simulink model "Lights_harness"  (Simulink 7.7)
settings: Solver=FixedStepDiscrete  SolverMode=SingleTasking  StartTime=0.0  StopTime=100  FixedStep=.01  RelTol=1e-3
PostLoadFcn:
  | cd '..';
  | PostLoadFcn;
  | cd 'harness';
InitFcn:
  | if signalbuilder('Lights_harness/Signal Builder','activegroup') == 1
  |   CD_LIGHTS_FUNCTION.DataType = 'uint8';
  |   CD_LIGHTS_FUNCTION.Value = 255;
  |   CD_LIGHTS_FEEDBACK_FUNCTION.DataType = 'uint8';
  |   CD_LIGHTS_FEEDBACK_FUNCTION.Value = 255;
  | else
  |   CD_LIGHTS_FUNCTION.DataType = 'uint8';
  |   CD_LIGHTS_FUNCTION.Value = 0;
  |   CD_LIGHTS_FEEDBACK_FUNCTION.DataType = 'uint8';
  |   CD_LIGHTS_FEEDBACK_FUNCTION.Value = 0;
  | end
undefined symbols (not defined in the file): ACTIVE, INACTIVE, LIGHT_BUTTON_MASK, LIGHT_BUTTON_PRESS, LOW, NO_COMMUNICATION, NON_FUNCTIONAL, NORMAL, OORL, sigbuilder_block, srate100
libraries: simulink x2, MX_Library x1
settings Model: Creator=smindema  LastModifiedBy=aliebel  CovMetricSettings=dcmw  CovHTMLOptions=-aTS=1 -bRG=1 -bTC=1 -hTR=0 -nFC=0 -scm=1 -bcm=1 -xEv=0  covSaveCumulativeToWorkspaceVar=off  CovSaveSingleToWorkspaceVar=off
settings MATStruct: SampleTime=0.01  Offset=0  Priority=[1.0]
settings DataIOCC: LimitDataPoints=off  SaveOutput=off  SaveTime=off
settings OptimizationCC: BlockReduction=off  InlineParams=on  ExpressionFolding=off  StateBitsets=on  DataBitsets=on  UseTempVars=on  InitFltsAndDblsToZero=on  NoFixptDivByZeroProtection=on  EfficientFloat2IntCast=on  OptimizeModelRefInitCode=on
settings DebuggingCC: SaveWithParameterizedLinksMsg=none  MultiTaskDSMMsg=warning  MultiTaskCondExecSysMsg=none  IntegerOverflowMsg=none  ModelReferenceCSMismatchMessage=warning
settings HardwareCC: ProdBitPerInt=16  ProdBitPerPointer=16  ProdIntDivRoundTo=Floor  ProdEndianess=BigEndian  ProdWordSize=16  ProdHWDeviceType=Motorola HC12
settings ModelReferenceCC: ModelReferenceNumInstancesAllowed=Single
settings RTWCC: SystemTargetFile=ert.tlc  GenCodeOnly=on  TemplateMakefile=ert_default_tmf  Description=Real-Time Workshop Embedded Coder (no auto configuration)  GenerateReport=on  RetainRTWFile=on  ProcessScript=ert_make_rtw_hook  IncludeHyperlinkInReport=on  LaunchReport=on  IncludeERTFirstTime=on
settings RTWCC: CustomHeaderCode=|
  | #include "cpp_req_defines.h"
  | #include "hw_fin.h"
  | #include "cdata.h"
settings CodeAppCC: IgnoreCustomStorageClasses=off  DefineNamingRule=UpperCase
settings ERTTargetCC: TargetFcnLib=ansi_tfl_tmw.mat  FunctionExecutionProfile=off  MultiwordLength=2048  GenerateSampleERTMain=on  IncludeMdlTerminateFcn=off  SupportAbsoluteTime=off  SupportNonFinite=off  SupportComplex=off  PurelyIntegerCode=on  ERTCustomFileTemplate=gen_rtw_req_defines_h.tlc  GlobalDataDefinition=InSeparateSourceFile  GlobalDataReference=InSeparateHeaderFile  ConvertIfToSwitch=off

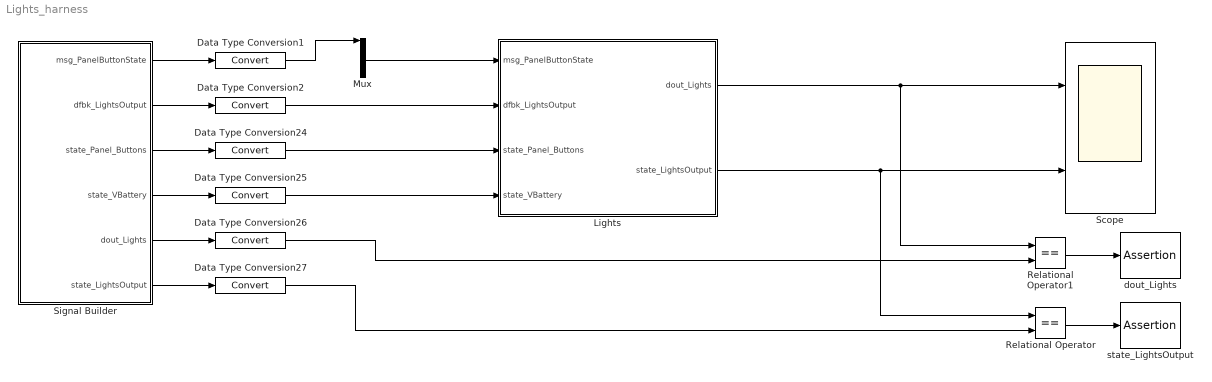
== system Lights_harness ==
  Data Type Conversion{1..2,24..27} (6 alike) : DataTypeConversion
  Lights : Subsystem  TreatAsAtomicUnit=on  SystemSampleTime=srate100  RTWFileName=mod_Outputs
      settings: RTWSystemCode=Function  RTWFileNameOpts=User specified
  Mux : Mux  Inputs=8
  Relational Operator : RelationalOperator  Operator===  OutDataTypeStr=boolean
  Relational Operator1 : RelationalOperator  Operator===  OutDataTypeStr=boolean
  Scope : Scope  NumInputPorts=2
      settings: TimeRange=100  YMin=0~0  YMax=6~10  DataFormat=Array
  Signal Builder : Subsystem  Tag=STV Subsys  LoadFcn=sigbuilder_block('load');  StartFcn=sigbuilder_block('start');  StopFcn=sigbuilder_block('stop');  ClipboardFcn=sigbuilder_block('clipboard');  mask(Sigbuilder block){}
      mask help: Create and generate interchangeable groups of signals whose waveforms are piecewise linear.
      mask init:
      | if ~strcmp(get_param(bdroot(gcbh),'SimulationStatus'),'stopped') tuvar = sigbuilder_block('maskInit'); end
      settings: CopyFcn=sigbuilder_block('copy');  DeleteFcn=sigbuilder_block('delete');  ModelCloseFcn=sigbuilder_block('modelClose');  PreSaveFcn=sigbuilder_block('preSave');  NameChangeFcn=sigbuilder_block('namechange');  OpenFcn=sigbuilder_block('open',[294.75 262.5 911.25 399.75 ]);  CloseFcn=sigbuilder_block('close');
      mask Display: plot(0, 0, 100, 100,[2, 2, 32, 32, 2], [68, 8, 8, 68, 68],[32, 2], [38, 38], [32, 19, 2],[53, 60, 44], [32, 17, 17, 2],[16, 16, 31, 31]);txt = getActiveGroup(gcbh);text(2, 100, txt,'verticalAlignment', 'top');
  dout_Lights : Assertion  Enabled=off
  state_LightsOutput : Assertion  Enabled=off
  wires:
  Relational Operator/1 -> state_LightsOutput/1
  Relational Operator1/1 -> dout_Lights/1
  Data Type Conversion26/1 -> Relational Operator1/2
  Data Type Conversion27/1 -> Relational Operator/2
  Lights/1(dout_Lights) -> Scope/1, Relational Operator1/1
  Lights/2(state_LightsOutput) -> Scope/2, Relational Operator/1
  Data Type Conversion2/1 -> Lights/2(dfbk_LightsOutput)
  Data Type Conversion24/1 -> Lights/3(state_Panel_Buttons)
  Data Type Conversion25/1 -> Lights/4(state_VBattery)
  Signal Builder/1(msg_PanelButtonState) -> Data Type Conversion1/1
  Signal Builder/2(dfbk_LightsOutput) -> Data Type Conversion2/1
  Signal Builder/3(state_Panel_Buttons) -> Data Type Conversion24/1
  Signal Builder/4(state_VBattery) -> Data Type Conversion25/1
  Signal Builder/5(dout_Lights) -> Data Type Conversion26/1
  Signal Builder/6(state_LightsOutput) -> Data Type Conversion27/1
  Mux/1 -> Lights/1(msg_PanelButtonState)
  Data Type Conversion1/1 -> Mux/1

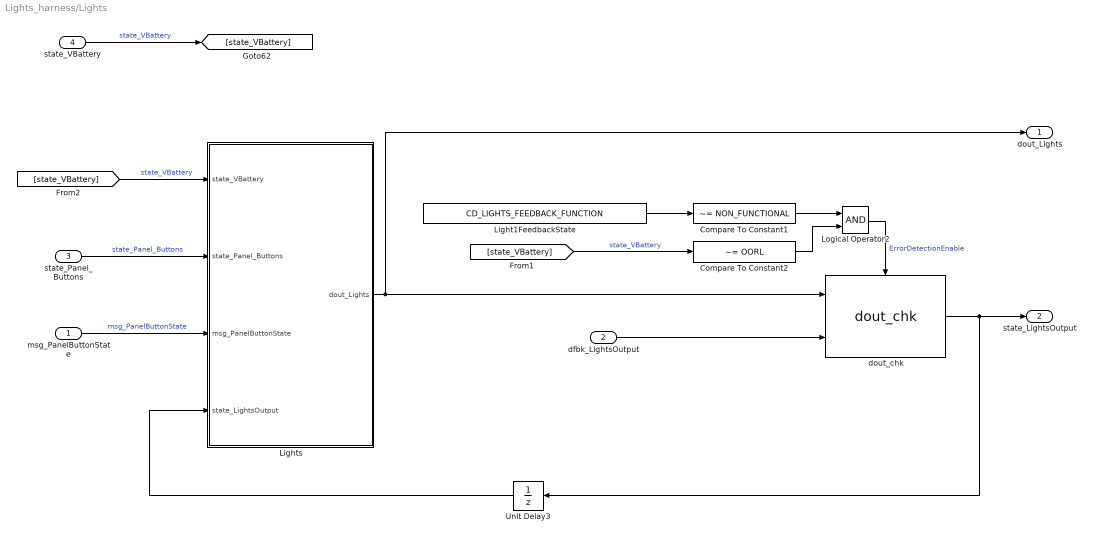
== system Lights_harness/Lights ==
  msg_PanelButtonState : Inport
  dfbk_LightsOutput : Inport  Port=2  OutDataTypeStr=boolean
  state_Panel_Buttons : Inport  Port=3  OutDataTypeStr=uint8
  state_VBattery : Inport  Port=4  OutDataTypeStr=uint8
  Compare To Constant1 : simulink/Logic and Bit Operations/Compare To Constant  SystemSampleTime=-1  relop=~=  const=NON_FUNCTIONAL  LogicOutDataTypeMode=boolean  ZeroCross=off
  Compare To Constant2 : simulink/Logic and Bit Operations/Compare To Constant  SystemSampleTime=-1  relop=~=  const=OORL  LogicOutDataTypeMode=boolean  ZeroCross=off
  Light1FeedbackState : Constant  Value=CD_LIGHTS_FEEDBACK_FUNCTION  OutDataTypeStr=uint8
  Lights : Stateflow chart  TreatAsAtomicUnit=on
  Logical Operator2 : Logic  AllPortsSameDT=off  OutDataTypeStr=boolean
  Unit Delay3 : UnitDelay  X0=NORMAL  SampleTime=-1
      settings: AttributesFormatString=<initial=%<X0>>\n<tsample=%<SampleTime>>
  dout_chk : MX_Library/dout_chk  SystemSampleTime=-1  ERR_ON_DB_CNT=CD_LIGHTS_DEBOUNCE_ERROR_ON  ERR_OFF_DB_CNT=CD_LIGHTS_DEBOUNCE_ERROR_OFF
  dout_Lights : Outport
  state_LightsOutput : Outport  Port=2
  wires:
  Lights/1(dout_Lights) -> dout_Lights/1, dout_chk/1
  [state_VBattery] -> Lights/1(state_VBattery)  "state_VBattery"
  dfbk_LightsOutput/1 -> dout_chk/2
  dout_chk/1 -> state_LightsOutput/1, Unit Delay3/1
  state_VBattery/1 -> [state_VBattery]  "state_VBattery"
  Logical Operator2/1 -> dout_chk/Enable  "ErrorDetectionEnable"
  Light1FeedbackState/1 -> Compare To Constant1/1
  [state_VBattery] -> Compare To Constant2/1  "state_VBattery"
  Compare To Constant1/1 -> Logical Operator2/1
  Compare To Constant2/1 -> Logical Operator2/2
  state_Panel_Buttons/1 -> Lights/2(state_Panel_Buttons)  "state_Panel_Buttons"
  Unit Delay3/1 -> Lights/4(state_LightsOutput)
  msg_PanelButtonState/1 -> Lights/3(msg_PanelButtonState)  "msg_PanelButtonState"

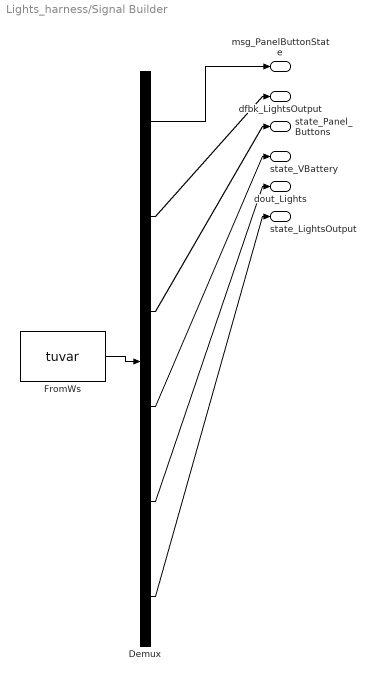
== system Lights_harness/Signal Builder ==
  Demux : Demux  Tag=STV Demux  Outputs=6
  FromWs : FromWorkspace  Tag=STV FromWs  VariableName=tuvar  SampleTime=0  SigBuilderData=DataTag0  VnvData=DataTag1
      SigBuilderData=|
      | common.afterFinalStr = 'Extrapolate'
      | common.sampleTime = 0
      | dataSet(1).timeRange = [0 100]
      | dataSet(1).name = 'NonFunctional'
      | dataSet(2).timeRange = [0 100]
      | dataSet(2).name = 'Functional'
      | sbobj.Groups(1).Name = 'NonFunctional'
      | sbobj.Groups(1).Signals(1).Name = 'msg_PanelButtonState'
      | sbobj.Groups(1).Signals(1).XData = [0 1 1 2 2 4 4 5 5 7 7 8 8 10 10 11 11 13 13 14 14 16 16 17 17 19 19 20 20 22 22 23 23 25 25 26 26 28 28 29 29 31 31 32 32 34 34 35 35 37 37 38 38 40 40 41 41 43 43 44 44 46 46 47 47 49 49 50 50 52 52 53 53 55 55 56 56 58 58 59 59 61 61 62 62 64 64 65 65 67 67 68 68 70 70 71 71 73 73 74 74 100]
      | sbobj.Groups(1).Signals(1).YData = [0 0 1 1 0 0 1 1 0 0 1 1 0 0 1 1 0 0 1 1 0 0 1 1 0 0 1 1 0 0 1 1 0 0 1 1 0 0 1 1 0 0 1 1 0 0 1 1 0 0 1 1 0 0 1 1 0 0 1 1 0 0 1 1 0 0 1 1 0 0 1 1 0 0 1 1 0 0 1 1 0 0 1 1 0 0 1 1 0 0 1 1 0 0 1 1 0 0 1 1 0 0]
      | sbobj.Groups(1).Signals(2).Name = 'dfbk_LightsOutput'
      | sbobj.Groups(1).Signals(2).XData = [0 18 18 36 36 54 54 72 72 100]
      | sbobj.Groups(1).Signals(2).YData = [0 0 1 1 0 0 1 1 0 0]
      | sbobj.Groups(1).Signals(3).Name = 'state_Panel_Buttons'
      | sbobj.Groups(1).Signals(3).XData = [0 9 9 18 18 27 27 36 36 45 45 54 54 63 63 72 81 100]
      | sbobj.Groups(1).Signals(3).YData = [8 8 4 4 8 8 4 4 8 8 4 4 8 8 4 4 4 4]
      | sbobj.Groups(1).Signals(4).Name = 'state_VBattery'
      | sbobj.Groups(1).Signals(4).XData = [0 3 3 6 6 9 9 12 12 15 15 18 18 21 21 24 24 27 27 30 30 33 33 36 36 39 39 42 42 45 45 48 48 51 51 54 54 57 57 60 60 63 63 66 66 69 69 72 72 100]
      | sbobj.Groups(1).Signals(4).YData = [8 8 9 9 14 14 8 8 9 9 14 14 8 8 9 9 14 14 8 8 9 9 14 14 8 8 9 9 14 14 8 8 9 9 14 14 8 8 9 9 14 14 8 8 9 9 14 14 8 8]
      | sbobj.Groups(1).Signals(5).Name = 'dout_Lights'
      | sbobj.Groups(1).Signals(5).XData = [0 100]
      | sbobj.Groups(1).Signals(5).YData = [0 0]
      | sbobj.Groups(1).Signals(6).Name = 'state_LightsOutput'
      | sbobj.Groups(1).Signals(6).XData = [0 100]
      | sbobj.Groups(1).Signals(6).YData = [8 8]
      | sbobj.Groups(1).TimeRange = [0 100]
      | sbobj.Groups(2).Name = 'Functional'
      | sbobj.Groups(2).Signals(1).Name = 'msg_PanelButtonState'
      | sbobj.Groups(2).Signals(1).XData = [0 1 1 2 2 4 4 5 5 7 7 8 8 10 10 11 11 13 13 14 14 20 20 21 21 31 31 32 32 43 43 44 44 52 52 53 53 70 70 71 71 73 73 75 75 100]
      | sbobj.Groups(2).Signals(1).YData = [0 0 1 1 0 0 1 1 0 0 1 1 0 0 1 1 0 0 1 1 0 0 1 1 0 0 1 1 0 0 1 1 0 0 1 1 0 0 1 1 0 0 1 1 0 0]
      | sbobj.Groups(2).Signals(2).Name = 'dfbk_LightsOutput'
      | sbobj.Groups(2).Signals(2).XData = [0 1 1 5 5 7 7 11 11 20 20 25 25 28.1 28.1 30.1 30.1 31.1 31.1 34.1 34.1 37 37 43 43 62 62 66 66 73 73 85.4 100]
      | sbobj.Groups(2).Signals(2).YData = [0 0 1 1 0 0 1 1 0 0 1 1 0 0 1 1 0 0 1 1 0 0 1 1 0 0 1 1 0 0 1 1 1]
      | sbobj.Groups(2).Signals(3).Name = 'state_Panel_Buttons'
      | sbobj.Groups(2).Signals(3).XData = [0 22 22 23 23 28 28 30 30 46 46 47 47 100]
      | sbobj.Groups(2).Signals(3).YData = [8 8 4 4 8 8 4 4 8 8 4 4 8 8]
      | sbobj.Groups(2).Signals(4).Name = 'state_VBattery'
      | sbobj.Groups(2).Signals(4).XData = [0 6 6 12 12 18 18 25 25 26 26 33 33 34 34 48 48 49 49 60 60 61 61 100]
      | sbobj.Groups(2).Signals(4).YData = [8 8 9 9 14 14 8 8 14 14 8 8 14 14 8 8 22 22 8 8 22 22 8 8]
      | sbobj.Groups(2).Signals(5).Name = 'dout_Lights'
      | sbobj.Groups(2).Signals(5).XData = [0 100]
      | sbobj.Groups(2).Signals(5).YData = [0 0]
      | sbobj.Groups(2).Signals(6).Name = 'state_LightsOutput'
      | sbobj.Groups(2).Signals(6).XData = [0 100]
      | sbobj.Groups(2).Signals(6).YData = [8 8]
      | sbobj.Groups(2).TimeRange = [0 100]
  msg_PanelButtonState : Outport  Tag=STV Outport
  dfbk_LightsOutput : Outport  Tag=STV Outport  Port=2
  state_Panel_Buttons : Outport  Tag=STV Outport  Port=3
  state_VBattery : Outport  Tag=STV Outport  Port=4
  dout_Lights : Outport  Tag=STV Outport  Port=5
  state_LightsOutput : Outport  Tag=STV Outport  Port=6
  wires:
  Demux/1 -> msg_PanelButtonState/1
  FromWs/1 -> Demux/1
  Demux/2 -> dfbk_LightsOutput/1
  Demux/3 -> state_Panel_Buttons/1
  Demux/4 -> state_VBattery/1
  Demux/5 -> dout_Lights/1
  Demux/6 -> state_LightsOutput/1

== stateflow chart Lights/Lights ==
  settings: executeAtInitialization=1
  state LIGHTS_INACTIVE
    en:
    dout_Lights = INACTIVE;
  state LIGHTS_ACTIVE
    en:
    state_Panel_Buttons_Old = state_Panel_Buttons;
    dout_Lights = ACTIVE;
  state LIGHTS_ACTIVE_RISING2
    en:
    dout_Lights = ACTIVE;
  state LIGHTS_ACTIVE_RISING1
    en:
    dout_Lights = ACTIVE;
  LIGHTS_ACTIVE -> LIGHTS_INACTIVE [order 1] : [(state_Panel_Buttons_Old == NO_COMMUNICATION)...
      | && (state_Panel_Buttons != NO_COMMUNICATION)...
      | || (!((state_VBattery == NORMAL) || (state_VBattery == LOW)))...
      | || (state_LightsOutput != NORMAL)]
  LIGHTS_INACTIVE -> LIGHTS_ACTIVE_RISING1 [order 2] : [((state_VBattery == NORMAL) || (state_VBattery == LOW))...
      | && (CD_LIGHTS_FUNCTION != NON_FUNCTIONAL)...
      | && ((msg_PanelButtonState[0] & LIGHT_BUTTON_MASK) == LIGHT_BUTTON_PRESS)...
      | && (state_LightsOutput == NORMAL)]
  LIGHTS_ACTIVE -> LIGHTS_ACTIVE_RISING2 [order 2] : [((msg_PanelButtonState[0] & LIGHT_BUTTON_MASK) == LIGHT_BUTTON_PRESS)]
  (default) -> LIGHTS_INACTIVE
  LIGHTS_ACTIVE_RISING2 -> LIGHTS_INACTIVE : [((msg_PanelButtonState[0] & LIGHT_BUTTON_MASK) == INACTIVE)]
  LIGHTS_ACTIVE_RISING1 -> LIGHTS_ACTIVE : [((msg_PanelButtonState[0] & LIGHT_BUTTON_MASK) == INACTIVE)]
  LIGHTS_INACTIVE -> LIGHTS_ACTIVE [order 1] : [(CD_LIGHTS_FUNCTION != NON_FUNCTIONAL)...
      | && (state_Panel_Buttons == NO_COMMUNICATION)...
      | && (state_LightsOutput == NORMAL)]
  data: state_VBattery input uint8; dout_Lights output boolean; ACTIVE parameter uint8 =1; LOW parameter uint8 =9; NORMAL parameter uint8 =8; INACTIVE parameter uint8 =0; CD_LIGHTS_FUNCTION parameter uint8 =8; state_Panel_Buttons input uint8; NO_COMMUNICATION parameter uint8; state_Panel_Buttons_Old local uint8; msg_PanelButtonState input uint8 size=8; LIGHT_BUTTON_MASK parameter uint8; LIGHT_BUTTON_PRESS parameter uint8; NON_FUNCTIONAL parameter uint8; state_LightsOutput input uint8
